simulink model "lalala"  (R2022a)
settings: Solver=VariableStepAuto  StartTime=0.0  StopTime=10.0  RelTol=1e-3
values from neighbouring files (symbols this model uses):
  c_bar = 4.9    [FinalProject.m]
  C_DM = 0.0223    [FinalProject.m]
  CL_0 = 0.307    [FinalProject.m]
  CL_a = 4.41    [FinalProject.m]
  CL_ad = 1.7    [FinalProject.m]
  CL_DM = 0    [FinalProject.m]
  CL_el = 0.43    [FinalProject.m]
  CL_q = 3.9    [FinalProject.m]
  CM_0 = 0.04    [FinalProject.m]
  CM_a = -0.613    [FinalProject.m]
  CM_ad = -7.27    [FinalProject.m]
  CM_el = -1.122    [FinalProject.m]
  CM_q = -12.4    [FinalProject.m]
  e_T = 0    [FinalProject.m]
  el = 0.0278    [FinalProject.m]
  epsilon = 0    [FinalProject.m]
  eta = .7    (= 0.7)    [FinalProject.m]
  J_2 = 1346    [FinalProject.m]
  k = 0.0554    [FinalProject.m]
  m = W / g    (= 82.298136646)    [FinalProject.m]
  rho = 2.377e-3    (= 0.002377)    [FinalProject.m]
  S = 174    [FinalProject.m]
  th = 100    [FinalProject.m]
  W = 2650    [FinalProject.m]
  x = 0    [FinalProject.m]
undefined symbols (not defined in the file or in its folder): magnitude
settings Model: PacingRate=4  Creator=nickmondora  LastModifiedBy=nickmondora

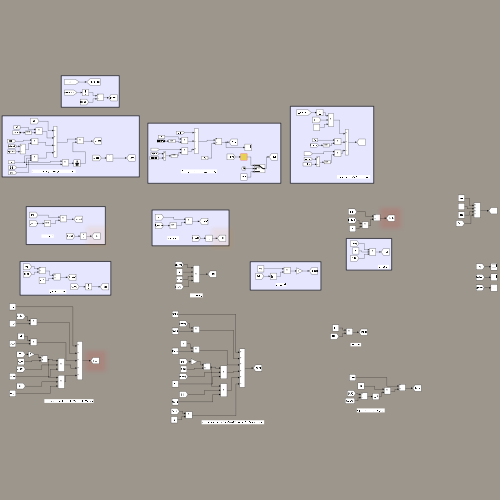
[thumbnail: Simulink's stored preview of the top-level diagram]
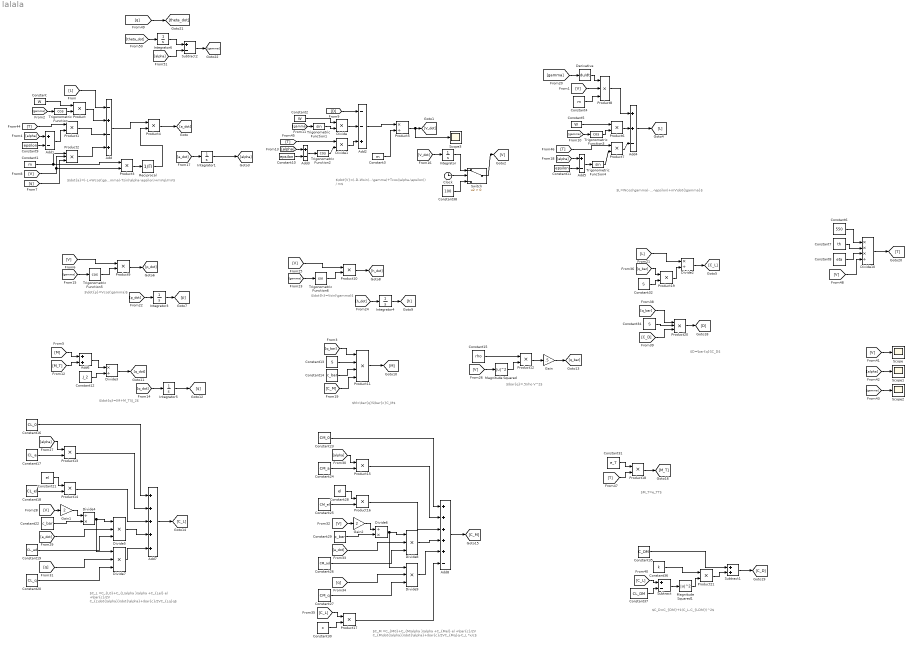
== system lalala ==
  note: $\dot{a}=(-L+Wcos(\gamma)-Tsin(\alpha-\epsilon)+mVq)/mV$
  note: $\dot{V}=(-D-Wsin(\gamma)+Tcos(\alpha-\epsilon)) / m$
  note: $\dot{p}=Vcos(\gamma)$
  note: $\dot{h}=Vsin(\gamma)$
  note: $\dot{q}=(M+M_T)/J_2$
  note: $M=\bar{q}S\bar{c}C_M$
  note: $\bar{q}=.5\rho V^2$
  note: $C_L =C_{L0}+C_{L\alpha }\alpha +C_{Lel} el +\bar{c}/2V C_{L\dot{\alpha}}\dot{\alpha}+\bar{c}/2VC_{Lq}q$
  note: $C_M =C_{M0}+C_{M\alpha }\alpha +C_{Mel} el +\bar{c}/2V C_{M\dot{\alpha}}\dot{\alpha}+\bar{c}/2VC_{Mq}q-C_L *x/c$
  note: $M_T=e_TT$
  note: $D=\bar{q}SC_D$
  note: $C_D=C_{DM}+k(C_L-C_{LDM})^2$
  note: $L=Wcos(\gamma)-Tsin(\alpha-\epsilon)+mV\dot{\gamma}$
  Add : Sum  Inputs=-+-+
  Add1 : Sum  Inputs=+-
  Add2 : Sum  Inputs=--+
  Add3 : Sum  Inputs=+-
  Add4 : Sum  Inputs=++-
  Add5 : Sum  Inputs=+-
  Add6 : Sum
  Add7 : Sum  Inputs=+++++
  Add8 : Sum  Inputs=+++++-
  Clock : Clock
  Constant : Constant  Value=W
  Constant1 : Constant  Value=m
  Constant10 : Constant  Value=epsilon
  Constant11 : Constant  Value=epsilon
  Constant12 : Constant  Value=J_2
  Constant13 : Constant  Value=S
  Constant14 : Constant  Value=c_bar
  Constant15 : Constant  Value=rho
  Constant16 : Constant  Value=CL_0
  Constant17 : Constant  Value=CL_a
  Constant18 : Constant  Value=CL_el
  Constant19 : Constant  Value=CL_ad
  Constant2 : Constant  Value=W
  Constant20 : Constant  Value=CL_q
  Constant21 : Constant  Value=el
  Constant22 : Constant  Value=c_bar
  Constant23 : Constant  Value=CM_0
  Constant24 : Constant  Value=CM_a
  Constant25 : Constant  Value=CM_el
  Constant26 : Constant  Value=CM_ad
  Constant27 : Constant  Value=CM_q
  Constant28 : Constant  Value=el
  Constant29 : Constant  Value=c_bar
  Constant3 : Constant  Value=m
  Constant30 : Constant  Value=x
  Constant31 : Constant  Value=e_T
  Constant32 : Constant  Value=S
  Constant34 : Constant  Value=S
  Constant35 : Constant  Value=C_DM
  Constant36 : Constant  Value=k
  Constant37 : Constant  Value=CL_DM
  Constant38 : Constant  Value=100
  Constant4 : Constant  Value=m
  Constant5 : Constant  Value=W
  Constant6 : Constant  Value=550
  Constant7 : Constant  Value=th
  Constant8 : Constant  Value=eta
  Constant9 : Constant  Value=epsilon
  Derivative : Derivative
  Divide : Product
  Divide1 : Product
  Divide10 : Product  Inputs=***/
  Divide2 : Product  Inputs=*/
  Divide3 : Product  Inputs=*/
  Divide4 : Product  Inputs=/*
  Divide{5,7..9} (4 alike) : Product  Inputs=***
  Divide6 : Product  Inputs=/*
  Gain : Gain  Gain=.5
  Gain1 : Gain  Gain=2
  Gain2 : Gain  Gain=2
  Integrator{,1,3..6} (6 alike) : Integrator
  Magnitude Squared : Math  Operator=magnitude^2
  Magnitude Squared1 : Math  Operator=magnitude^2
  Product{,1,3..4,6..7,9..10,12..19,21} (17 alike) : Product
  Product11 : Product  Inputs=4
  Product2 : Product  Inputs=3
  Product20 : Product  Inputs=3
  Product5 : Product  Inputs=*/
  Product8 : Product  Inputs=3
  Reciprocal : Product  Inputs=/
  Scope{,1..3} (4 alike) : Scope
  Subtract : Sum  Inputs=+-
  Subtract1 : Sum
  Subtract2 : Sum  Inputs=+-
  Switch : Switch  Criteria=u2 > Threshold  SaturateOnIntegerOverflow=off  InputSameDT=off
  Trigonometric Function{,2..3,5} (4 alike) : Trigonometry  Operator=cos
  Trigonometric Function1 : Trigonometry
  Trigonometric Function4 : Trigonometry
  Trigonometric Function6 : Trigonometry
  wires:
  [L] -> Add/1
  [gamma] -> Trigonometric Function/1
  Trigonometric Function/1 -> Product/2
  Constant/1 -> Product/1
  Product/1 -> Add/2
  [alpha] -> Add1/1
  Constant9/1 -> Add1/2
  Product1/1 -> Add/3
  [T] -> Product1/1
  Add1/1 -> Product1/2
  Product2/1 -> Add/4
  Constant1/1 -> Product3/1, Product2/1
  [V] -> Product3/2, Product2/2
  [q] -> Product2/3
  Product3/1 -> Reciprocal/1
  Add/1 -> Product4/1
  Reciprocal/1 -> Product4/2
  Product4/1 -> [a_dot]
  [D] -> Add2/1
  [gamma] -> Trigonometric Function1/1
  Divide/1 -> Add2/2
  Constant2/1 -> Divide/1
  Trigonometric Function1/1 -> Divide/2
  [alpha] -> Add3/1
  Constant10/1 -> Add3/2
  Add3/1 -> Trigonometric Function2/1
  Trigonometric Function2/1 -> Divide1/2
  [T] -> Divide1/1
  Divide1/1 -> Add2/3
  Constant3/1 -> Product5/2
  Add2/1 -> Product5/1
  Product5/1 -> Scope3/1, [V_dot]
  [V_dot] -> Integrator/1
  [a_dot] -> Integrator1/1
  Integrator1/1 -> [alpha]
  [gamma] -> Trigonometric Function3/1
  Product6/1 -> Add4/2
  Constant5/1 -> Product6/1
  Trigonometric Function3/1 -> Product6/2
  [alpha] -> Add5/1
  Constant11/1 -> Add5/2
  Add5/1 -> Trigonometric Function4/1
  Product7/1 -> Add4/3
  [T] -> Product7/1
  Trigonometric Function4/1 -> Product7/2
  [gamma] -> Trigonometric Function5/1
  [V] -> Product9/1
  Trigonometric Function5/1 -> Product9/2
  Product9/1 -> [p_dot]
  [p_dot] -> Integrator3/1
  Integrator3/1 -> [p]
  [gamma] -> Trigonometric Function6/1
  [h_dot] -> Integrator4/1
  Integrator4/1 -> [h]
  Trigonometric Function6/1 -> Product10/2
  Product10/1 -> [h_dot]
  [V] -> Product10/1
  [M] -> Add6/1
  [M_T] -> Add6/2
  Add6/1 -> Divide3/1
  Constant12/1 -> Divide3/2
  [q_dot] -> Integrator5/1
  Divide3/1 -> [q_dot]
  Integrator5/1 -> [q]
  [q_bar] -> Product11/1
  Constant13/1 -> Product11/2
  Constant14/1 -> Product11/3
  [C_M] -> Product11/4
  Product11/1 -> [M]
  [V] -> Magnitude Squared/1
  Constant15/1 -> Product12/1
  Magnitude Squared/1 -> Product12/2
  Product12/1 -> Gain/1
  Gain/1 -> [q_bar]
  [alpha] -> Product13/1
  Constant17/1 -> Product13/2
  Constant18/1 -> Product14/2
  Constant21/1 -> Product14/1
  [V] -> Gain1/1
  Gain1/1 -> Divide4/1
  Constant22/1 -> Divide4/2
  Divide4/1 -> Divide7/1, Divide5/1
  [a_dot] -> Divide5/2
  Constant19/1 -> Divide5/3
  [q] -> Divide7/2
  Constant20/1 -> Divide7/3
  Divide5/1 -> Add7/4
  Divide7/1 -> Add7/5
  Product14/1 -> Add7/3
  Product13/1 -> Add7/2
  Add7/1 -> [C_L]
  Divide8/1 -> Add8/4
  Product16/1 -> Add8/3
  [alpha] -> Product15/1
  [V] -> Gain2/1
  Constant29/1 -> Divide6/2
  Constant25/1 -> Product16/2
  Product15/1 -> Add8/2
  Constant28/1 -> Product16/1
  Divide6/1 -> Divide9/1, Divide8/1
  Add8/1 -> [C_M]
  Divide9/1 -> Add8/5
  Constant26/1 -> Divide8/3
  [a_dot] -> Divide8/2
  Gain2/1 -> Divide6/1
  Constant24/1 -> Product15/2
  Constant27/1 -> Divide9/3
  [q] -> Divide9/2
  [C_L] -> Product17/1
  Constant30/1 -> Product17/2
  Product17/1 -> Add8/6
  Constant23/1 -> Add8/1
  Constant16/1 -> Add7/1
  Constant31/1 -> Product18/1
  [T] -> Product18/2
  Product18/1 -> [M_T]
  Product20/1 -> [D]
  Constant34/1 -> Product20/2
  [q_bar] -> Product20/1
  [C_D] -> Product20/3
  [C_L] -> Subtract/1
  Constant37/1 -> Subtract/2
  Subtract/1 -> Magnitude Squared1/1
  Magnitude Squared1/1 -> Product21/2
  Constant36/1 -> Product21/1
  Product21/1 -> Subtract1/2
  Constant35/1 -> Subtract1/1
  Subtract1/1 -> [C_D]
  [V] -> Scope/1
  [alpha] -> Scope1/1
  [gamma] -> Scope2/1
  Switch/1 -> [V]
  Integrator/1 -> Switch/1
  Clock/1 -> Switch/2
  Constant38/1 -> Switch/3
  Constant6/1 -> Divide10/1
  Constant7/1 -> Divide10/2
  Constant8/1 -> Divide10/3
  [V] -> Divide10/4
  Divide10/1 -> [T]
  [q] -> [theta_dot]
  [theta_dot] -> Integrator6/1
  [alpha] -> Subtract2/2
  Integrator6/1 -> Subtract2/1
  Subtract2/1 -> [gamma]
  [V] -> Product8/2
  Constant4/1 -> Product8/3
  Product8/1 -> Add4/1
  Add4/1 -> [L]
  [gamma] -> Derivative/1
  Derivative/1 -> Product8/1
  [q_bar] -> Product19/1
  Constant32/1 -> Product19/2
  [L] -> Divide2/1
  Product19/1 -> Divide2/2
  Divide2/1 -> [C_L]
